simulink model "formation2"  (Simulink 6.6)
settings: Solver=ode45  StartTime=0.0  StopTime=10.0  RelTol=1e-3
settings Model: Creator=wizest  LastModifiedBy=wizest

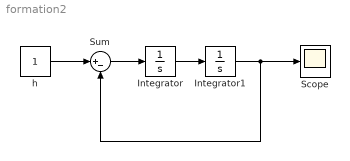
== system formation2 ==
  Integrator : Integrator
  Integrator1 : Integrator
  Scope : Scope
      settings: TimeRange=10  YMin=0  YMax=2
  Sum : Sum  Inputs=|+-
  h : Constant
  wires:
  Integrator/1 -> Integrator1/1
  Integrator1/1 -> Sum/2, Scope/1
  Sum/1 -> Integrator/1
  h/1 -> Sum/1
